simulink model "PMSM_Test_Bench"  (R2020a)
settings: Solver=VariableStepAuto  StartTime=0.0  StopTime=10.0  RelTol=1e-3  EnableMultiTasking=on
model workspace (MAT data in the model file):
  B = 0
  J = 5e-06
  KC = 0.04
  KV = 0.021
  L = 0.00021
  PP = 3
  R = 0.215
settings Model: Creator=admin_aboyer  LastModifiedBy=a_boyer
settings DataIOCC: ReturnWorkspaceOutputs=off
settings OptimizationCC: LifeSpan=inf
settings DebuggingCC: SFUnexpectedBacktrackingDiag=warning  SFNoUnconditionalDefaultTransitionDiag=warning  ArithmeticOperatorsInVariantConditions=warning
settings SFSimCC: SimUseLocalCustomCode=off  CustomCodeUndefinedFunction=UseInterfaceOnly
settings RTWCC: RTWUseLocalCustomCode=off
settings CodeAppCC: StateflowObjectComments=on
settings GRTTargetCC: TargetLangStandard=C89/C90 (ANSI)
settings ConfigComp: CovMetricSettings=dw  CovHtmlReporting=on  CovSaveCumulativeToWorkspaceVar=on  CovSaveSingleToWorkspaceVar=on  CovExternalEMLEnable=off

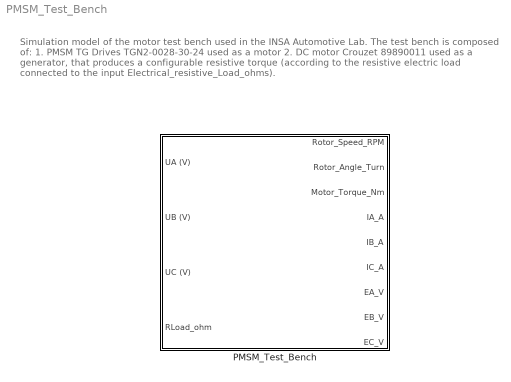
== system PMSM_Test_Bench ==
  note: Simulation model of the motor test bench used in the INSA Automotive Lab.
      | The test bench is composed of:
      | 1. PMSM TG Drives TGN2-0028-30-24 used as a motor
      | 2. DC motor Crouzet 89890011 used as a generator, that produces a configurable resistive torque
      | (according to the resistive electric load connected to the input Electrical_resistive_Load_ohms).
  PMSM_Test_Bench : Subsystem

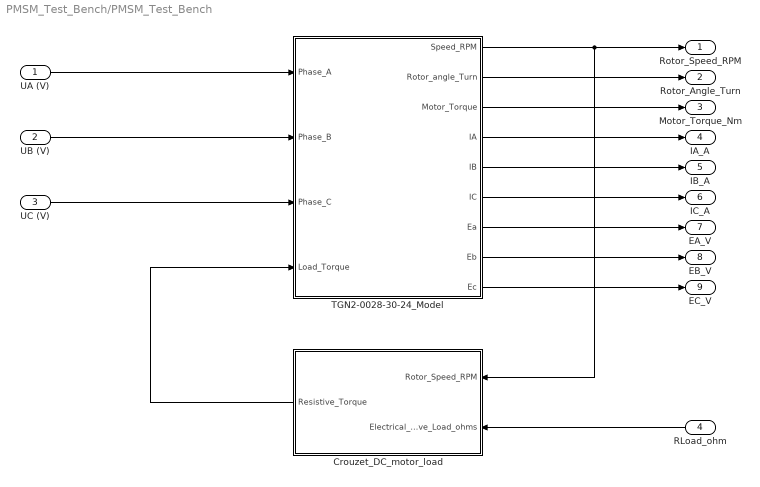
== system PMSM_Test_Bench/PMSM_Test_Bench ==
  UA (V) : Inport
  UB (V) : Inport  Port=2
  UC (V) : Inport  Port=3
  RLoad_ohm : Inport  Port=4
  Crouzet_DC_motor_load : Subsystem
  TGN2-0028-30-24_Model : Subsystem
      mask Display: image('C:\WORKSPACE_MATLAB\PMSM_Workshop\M5\img\PMSM.PNG');
  Rotor_Speed_RPM : Outport
  Rotor_Angle_Turn : Outport  Port=2
  Motor_Torque_Nm : Outport  Port=3
  IA_A : Outport  Port=4
  IB_A : Outport  Port=5
  IC_A : Outport  Port=6
  EA_V : Outport  Port=7
  EB_V : Outport  Port=8
  EC_V : Outport  Port=9
  wires:
  Crouzet_DC_motor_load/1(Resistive_Torque) -> TGN2-0028-30-24_Model/4(Load_Torque)
  TGN2-0028-30-24_Model/1(Speed_RPM) -> Rotor_Speed_RPM/1, Crouzet_DC_motor_load/1(Rotor_Speed_RPM)
  UA (V)/1 -> TGN2-0028-30-24_Model/1(Phase_A)
  UB (V)/1 -> TGN2-0028-30-24_Model/2(Phase_B)
  UC (V)/1 -> TGN2-0028-30-24_Model/3(Phase_C)
  TGN2-0028-30-24_Model/2(Rotor_angle_Turn) -> Rotor_Angle_Turn/1
  TGN2-0028-30-24_Model/3(Motor_Torque) -> Motor_Torque_Nm/1
  TGN2-0028-30-24_Model/4(IA) -> IA_A/1
  TGN2-0028-30-24_Model/5(IB) -> IB_A/1
  TGN2-0028-30-24_Model/6(IC) -> IC_A/1
  TGN2-0028-30-24_Model/7(Ea) -> EA_V/1
  TGN2-0028-30-24_Model/8(Eb) -> EB_V/1
  TGN2-0028-30-24_Model/9(Ec) -> EC_V/1
  RLoad_ohm/1 -> Crouzet_DC_motor_load/2(Electrical_resistive_Load_ohms)

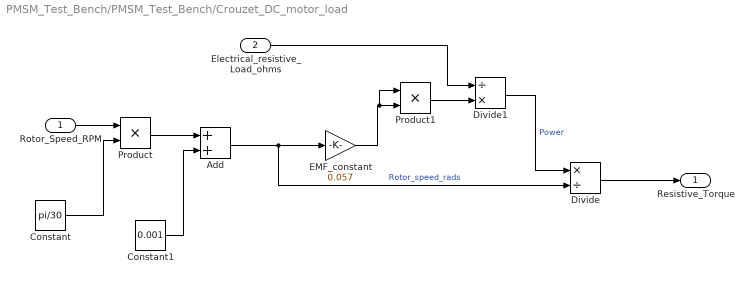
== system PMSM_Test_Bench/PMSM_Test_Bench/Crouzet_DC_motor_load ==
  Rotor_Speed_RPM : Inport
  Electrical_resistive_Load_ohms : Inport  Port=2
  Add : Sum
  Constant : Constant  Value=pi/30
  Constant1 : Constant  Value=0.001
  Divide : Product  Inputs=*/
  Divide1 : Product  Inputs=/*
  EMF_constant : Gain  Gain=0.057
  Product : Product
  Product1 : Product
  Resistive_Torque : Outport
  wires:
  Rotor_Speed_RPM/1 -> Product/1
  Constant/1 -> Product/2
  Product/1 -> Add/1
  Constant1/1 -> Add/2
  Add/1 -> Divide/2, EMF_constant/1  "Rotor_speed_rads"
  EMF_constant/1 -> Product1/1, Product1/2
  Product1/1 -> Divide1/2
  Divide1/1 -> Divide/1  "Power"
  Divide/1 -> Resistive_Torque/1
  Electrical_resistive_Load_ohms/1 -> Divide1/1

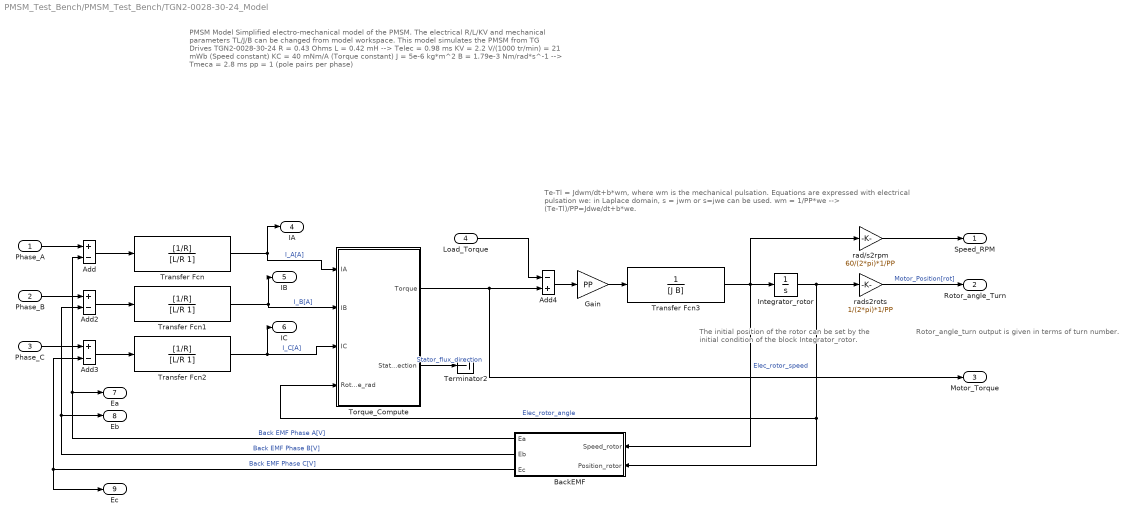
== system PMSM_Test_Bench/PMSM_Test_Bench/TGN2-0028-30-24_Model ==
  note: The initial position of the rotor can be set by the
      | initial condition of the block Integrator_rotor.
  note: Te-Tl = Jdwm/dt+b*wm, where wm is the mechanical pulsation.
      | Equations are expressed with electrical pulsation we: in Laplace domain, s = jwm or s=jwe can be used.
      | wm = 1/PP*we --> (Te-Tl)/PP=Jdwe/dt+b*we.
  note: PMSM Model
      |
      | Simplified electro-mechanical model of the PMSM. The electrical R/L/KV and mechanical parameters TL/J/B can be changed from model workspace.
      |
      | This model simulates the PMSM from TG Drives TGN2-0028-30-24
      | R = 0.43 Ohms
      | L = 0.42 mH --> Telec = 0.98 ms
      | KV = 2.2 V/(1000 tr/min) = 21 mWb (Speed constant)
      | KC = 40 mNm/A (Torque constant)
      | J = 5e-6 kg*m^2
      | B = 1.79e-3 Nm/rad*s^-1 --> Tmeca = 2.8 ms
      | pp = 1 (pole pairs per phase)
  note: Rotor_angle_turn output is given in terms of turn number.
  Phase_A : Inport
  Phase_B : Inport  Port=2
  Phase_C : Inport  Port=3
  Load_Torque : Inport  Port=4
  Add : Sum  Inputs=+-
  Add2 : Sum  Inputs=+-
  Add3 : Sum  Inputs=+-
  Add4 : Sum  Inputs=-+
  BackEMF : Subsystem
  Gain : Gain  Gain=PP
  Integrator_rotor : Integrator  InitialCondition=-pi/2
  Terminator2 : Terminator
  Torque_Compute : Subsystem
  Transfer Fcn : TransferFcn  Numerator=[1/R]  Denominator=[L/R 1]
  Transfer Fcn1 : TransferFcn  Numerator=[1/R]  Denominator=[L/R 1]
  Transfer Fcn2 : TransferFcn  Numerator=[1/R]  Denominator=[L/R 1]
  Transfer Fcn3 : TransferFcn  Denominator=[J B]
  rad/s2rpm : Gain  Gain=60/(2*pi)*1/PP
  rads2rots : Gain  Gain=1/(2*pi)*1/PP
  Speed_RPM : Outport
  Rotor_angle_Turn : Outport  Port=2
  Motor_Torque : Outport  Port=3
  IA : Outport  Port=4
  IB : Outport  Port=5
  IC : Outport  Port=6
  Ea : Outport  Port=7
  Eb : Outport  Port=8
  Ec : Outport  Port=9
  wires:
  Add/1 -> Transfer Fcn/1
  Phase_A/1 -> Add/1
  Transfer Fcn/1 -> Torque_Compute/1(IA), IA/1  "I_A[A]"
  Transfer Fcn1/1 -> IB/1, Torque_Compute/2(IB)  "I_B[A]"
  Add2/1 -> Transfer Fcn1/1
  Add3/1 -> Transfer Fcn2/1
  Transfer Fcn2/1 -> IC/1, Torque_Compute/3(IC)  "I_C[A]"
  Phase_B/1 -> Add2/1
  Phase_C/1 -> Add3/1
  Load_Torque/1 -> Add4/1
  Add4/1 -> Gain/1
  Gain/1 -> Transfer Fcn3/1
  Transfer Fcn3/1 -> BackEMF/1(Speed_rotor), Integrator_rotor/1, rad/s2rpm/1  "Elec_rotor_speed"
  Torque_Compute/1(Torque) -> Motor_Torque/1, Add4/2
  BackEMF/3(Ec) -> Add3/2, Ec/1  "Back EMF Phase C[V]"
  BackEMF/1(Ea) -> Ea/1, Add/2  "Back EMF Phase A[V]"
  BackEMF/2(Eb) -> Eb/1, Add2/2  "Back EMF Phase B[V]"
  rad/s2rpm/1 -> Speed_RPM/1
  Integrator_rotor/1 -> Torque_Compute/4(Rotor_angle_rad), BackEMF/2(Position_rotor), rads2rots/1  "Elec_rotor_angle"
  rads2rots/1 -> Rotor_angle_Turn/1  "Motor_Position[rot]"
  Torque_Compute/2(Stator_Flux_Direction) -> Terminator2/1  "Stator_flux_direction"

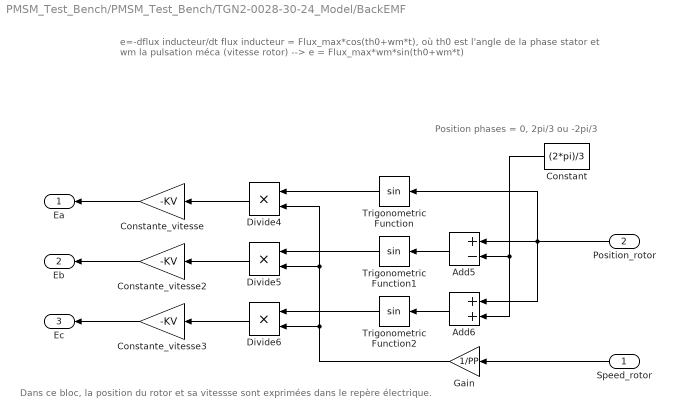
== system PMSM_Test_Bench/PMSM_Test_Bench/TGN2-0028-30-24_Model/BackEMF ==
  note: Dans ce bloc, la position du rotor et sa vitessse sont exprimées dans le repère électrique.
  note: e=-dflux inducteur/dt
      | flux inducteur = Flux_max*cos(th0+wm*t), où th0 est l'angle de la phase stator et wm la pulsation méca (vitesse rotor)
      | --> e = Flux_max*wm*sin(th0+wm*t)
  note: Position phases = 0, 2pi/3 ou -2pi/3
  Speed_rotor : Inport
  Position_rotor : Inport  Port=2
  Add5 : Sum  Inputs=+-
  Add6 : Sum
  Constant : Constant  Value=(2*pi)/3
  Constante_vitesse : Gain  Gain=-KV
  Constante_vitesse2 : Gain  Gain=-KV
  Constante_vitesse3 : Gain  Gain=-KV
  Divide4 : Product  Inputs=**
  Divide5 : Product  Inputs=**
  Divide6 : Product  Inputs=**
  Gain : Gain  Gain=1/PP
  Trigonometric Function : Trigonometry
  Trigonometric Function1 : Trigonometry
  Trigonometric Function2 : Trigonometry
  Ea : Outport
  Eb : Outport  Port=2
  Ec : Outport  Port=3
  wires:
  Divide4/1 -> Constante_vitesse/1
  Divide6/1 -> Constante_vitesse3/1
  Trigonometric Function2/1 -> Divide6/1
  Constante_vitesse3/1 -> Ec/1
  Speed_rotor/1 -> Gain/1
  Constante_vitesse2/1 -> Eb/1
  Divide5/1 -> Constante_vitesse2/1
  Constant/1 -> Add6/2, Add5/2
  Add6/1 -> Trigonometric Function2/1
  Trigonometric Function/1 -> Divide4/1
  Add5/1 -> Trigonometric Function1/1
  Constante_vitesse/1 -> Ea/1
  Trigonometric Function1/1 -> Divide5/1
  Position_rotor/1 -> Add5/1, Trigonometric Function/1, Add6/1
  Gain/1 -> Divide4/2, Divide5/2, Divide6/2

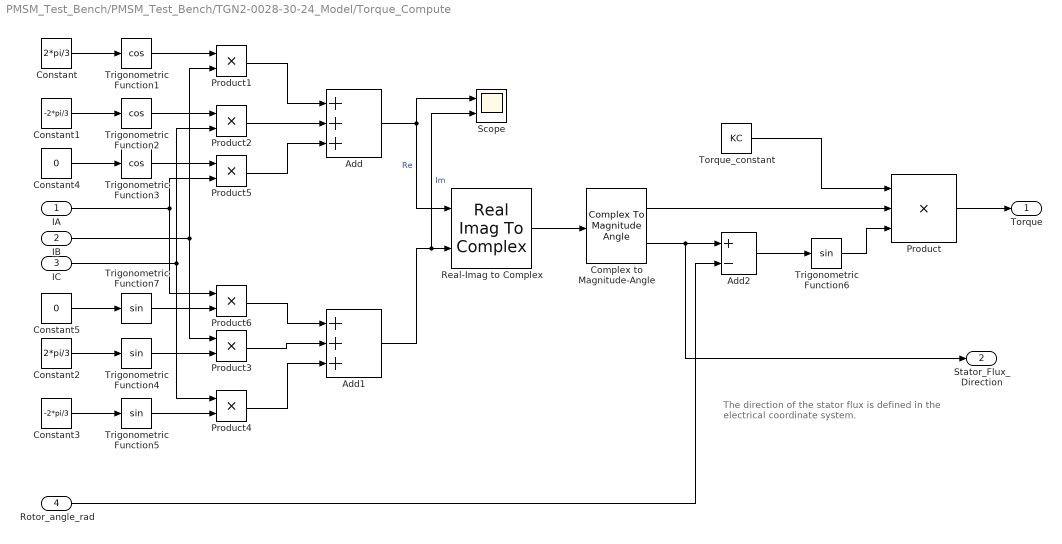
== system PMSM_Test_Bench/PMSM_Test_Bench/TGN2-0028-30-24_Model/Torque_Compute ==
  note: The direction of the stator flux is defined in the
      | electrical coordinate system.
  IA : Inport
  IB : Inport  Port=2
  IC : Inport  Port=3
  Rotor_angle_rad : Inport  Port=4
  Add : Sum  Inputs=+++
  Add1 : Sum  Inputs=+++
  Add2 : Sum  Inputs=+-
  Complex to Magnitude-Angle : ComplexToMagnitudeAngle
  Constant : Constant  Value=2*pi/3
  Constant1 : Constant  Value=-2*pi/3
  Constant2 : Constant  Value=2*pi/3
  Constant3 : Constant  Value=-2*pi/3
  Constant4 : Constant  Value=0
  Constant5 : Constant  Value=0
  Product : Product  Inputs=3
  Product{1..6} (6 alike) : Product
  Real-Imag to Complex : RealImagToComplex
  Scope : Scope  NumInputPorts=2
  Torque_constant : Constant  Value=KC
  Trigonometric Function1 : Trigonometry  Operator=cos
  Trigonometric Function2 : Trigonometry  Operator=cos
  Trigonometric Function3 : Trigonometry  Operator=cos
  Trigonometric Function{4..7} (4 alike) : Trigonometry
  Torque : Outport
  Stator_Flux_Direction : Outport  Port=2
  wires:
  Add/1 -> Real-Imag to Complex/1, Scope/1  "Re"
  Add1/1 -> Scope/2, Real-Imag to Complex/2  "Im"
  Real-Imag to Complex/1 -> Complex to Magnitude-Angle/1
  Complex to Magnitude-Angle/2 -> Stator_Flux_Direction/1, Add2/1
  Rotor_angle_rad/1 -> Add2/2
  Add2/1 -> Trigonometric Function6/1
  Complex to Magnitude-Angle/1 -> Product/2
  Trigonometric Function6/1 -> Product/3
  Torque_constant/1 -> Product/1
  Product/1 -> Torque/1
  Constant1/1 -> Trigonometric Function2/1
  Constant/1 -> Trigonometric Function1/1
  Trigonometric Function1/1 -> Product1/1
  Trigonometric Function2/1 -> Product2/1
  IB/1 -> Product1/2, Product3/1
  IC/1 -> Product4/1, Product2/2
  Product1/1 -> Add/1
  Product2/1 -> Add/2
  Constant3/1 -> Trigonometric Function5/1
  Constant2/1 -> Trigonometric Function4/1
  Trigonometric Function4/1 -> Product3/2
  Trigonometric Function5/1 -> Product4/2
  Product3/1 -> Add1/2
  Product4/1 -> Add1/3
  Constant4/1 -> Trigonometric Function3/1
  Trigonometric Function3/1 -> Product5/1
  IA/1 -> Product6/1, Product5/2
  Product5/1 -> Add/3
  Trigonometric Function7/1 -> Product6/2
  Constant5/1 -> Trigonometric Function7/1
  Product6/1 -> Add1/1
